simulink model "testmodel"  (R2016b)
settings: Solver=FixedStepDiscrete  StartTime=0.0  StopTime=10.0  RelTol=1e-3  EnableMultiTasking=on
libraries: frdmtfcshieldlib x5, simulink x3, frdmkl25zlib x2, etargetslib x1
settings Model: ExtModeTrigDuration=5  Creator=jays  LastModifiedBy=jays
settings OptimizationCC: MaxStackSize=64
settings DebuggingCC: ParameterTunabilityLossMsg=error
settings HardwareCC: ProdBitPerPointer=32  ProdBitPerSizeT=32  ProdBitPerPtrDiffT=32  ProdLargestAtomicInteger=Long  ProdLargestAtomicFloat=Double  ProdWordSize=32  ProdHWDeviceType=ARM Compatible->ARM Cortex
settings RTWCC: SystemTargetFile=ert.tlc  HardwareBoard=NXP FRDM-KL25Z  TLCOptions=-aInlineSetEventsForThisBaseRateFcn=TLC_FALSE -aSuppressMultiTaskScheduler=TLC_FALSE -aRateBasedStepFcn=1  TemplateMakefile=ert_default_tmf  Description=Embedded Coder  GenerateReport=on  Toolchain=GNU Tools for ARM Embedded Processors  IncludeHyperlinkInReport=on  LaunchReport=on  GenerateTraceInfo=on  GenerateTraceReport=on  GenerateTraceReportSl=on  GenerateTraceReportSf=on  GenerateTraceReportEml=on
settings CodeAppCC: ForceParamTrailComments=on  IgnoreCustomStorageClasses=off  OperatorAnnotations=on  SimulinkDataObjDesc=on  SFDataObjDesc=on  MATLABFcnDesc=on  InsertBlockDesc=on  MATLABSourceComments=on

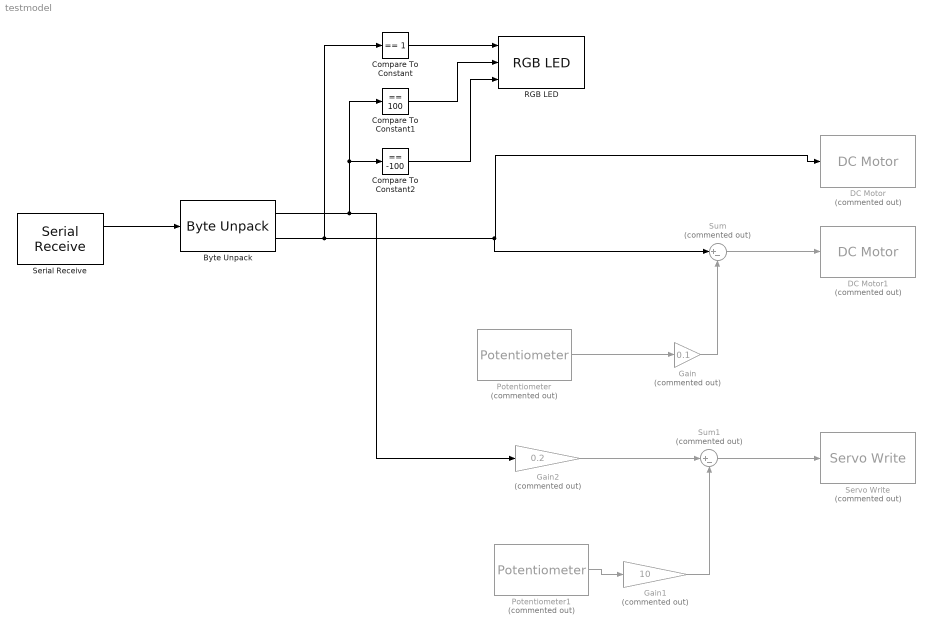
== system testmodel ==
  Byte Unpack : etargetslib/Byte Unpack  dimensions={[1],[1]}  datatypes={'int8','double'}  byteAlign=1
  Compare To Constant : simulink/Logic and Bit Operations/Compare To Constant  relop===  const=1  OutDataTypeStr=boolean
  Compare To Constant1 : simulink/Logic and Bit Operations/Compare To Constant  relop===  const=100  OutDataTypeStr=boolean
  Compare To Constant2 : simulink/Logic and Bit Operations/Compare To Constant  relop===  const=-100  OutDataTypeStr=boolean
  DC Motor : frdmtfcshieldlib/DC Motor  Commented=on  WhichMotor=A
  DC Motor1 : frdmtfcshieldlib/DC Motor  Commented=on  WhichMotor=B
  Gain : Gain  Commented=on  Gain=0.1
  Gain1 : Gain  Commented=on  Gain=10
  Gain2 : Gain  Commented=on  Gain=0.2
  Potentiometer : frdmtfcshieldlib/Potentiometer  Commented=on  WhichPot=A  SampleTime=0.0001
  Potentiometer1 : frdmtfcshieldlib/Potentiometer  Commented=on  WhichPot=B  SampleTime=0.0001
  RGB LED : frdmkl25zlib/RGB LED
  Serial Receive : frdmkl25zlib/Serial Receive  uart=UART0  DataType=uint8  DataLength=9  SampleTime=1
  Servo Write : frdmtfcshieldlib/Servo Write  Commented=on  WhichServo=0  minAngle=-20.0  maxAngle=20.0
  Sum : Sum  Commented=on  Inputs=|+-
  Sum1 : Sum  Commented=on  Inputs=|+-
  wires:
  Byte Unpack/1 -> Compare To Constant1/1, Compare To Constant2/1, Gain2/1
  Byte Unpack/2 -> Compare To Constant/1, Sum/1, DC Motor/1
  Potentiometer1/1 -> Gain1/1
  Gain1/1 -> Sum1/2
  Potentiometer/1 -> Gain/1
  Gain/1 -> Sum/2
  Sum1/1 -> Servo Write/1
  Gain2/1 -> Sum1/1
  Sum/1 -> DC Motor1/1
  Serial Receive/1 -> Byte Unpack/1
  Compare To Constant/1 -> RGB LED/1
  Compare To Constant1/1 -> RGB LED/2
  Compare To Constant2/1 -> RGB LED/3
